simulink subsystem "AS5600_Position_Sensor"  (R2022b)
settings: Solver=VariableStepAuto  StartTime=0.0  StopTime=10.0  RelTol=1e-3
libraries: dspsigops x1
settings Model: Creator=gotta  LastModifiedBy=gotta

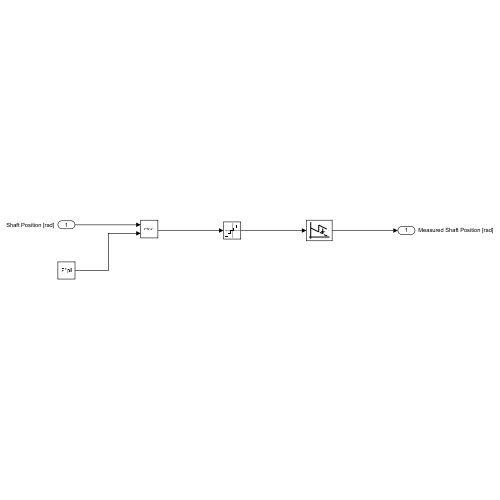
[thumbnail: Simulink's stored preview of the top-level diagram]
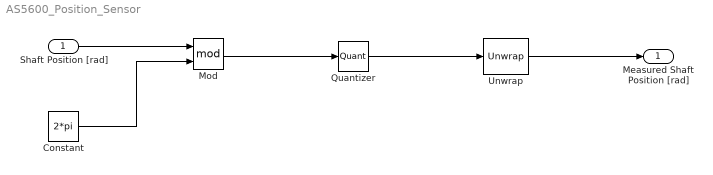
== system AS5600_Position_Sensor ==
  Shaft Position [rad] : Inport
  Constant : Constant  Value=2*pi
  Mod : Math  Operator=mod
  Quantizer : Quantizer  QuantizationInterval=AS5600.q_rad
  Unwrap : dspsigops/Unwrap  tol=pi  InputProcessing=Columns as channels (frame based)  running=off
  Measured Shaft Position [rad] : Outport
  wires:
  Shaft Position [rad]/1 -> Mod/1
  Constant/1 -> Mod/2
  Mod/1 -> Quantizer/1
  Quantizer/1 -> Unwrap/1
  Unwrap/1 -> Measured Shaft Position [rad]/1
